simulink model "lon_Input"  (R2016a)
settings: Solver=VariableStepAuto  StartTime=0.0  StopTime=1000  RelTol=1e-3
undefined symbols (not defined in the file): Alon, Blon, Clon, Dlon
settings Model: Creator=Gray  LastModifiedBy=Gray

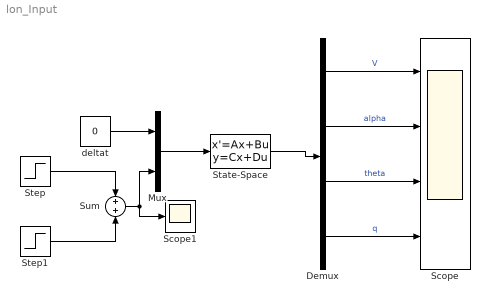
== system lon_Input ==
  Demux : Demux
  Mux : Mux  Inputs=2
  Scope : Scope  NumInputPorts=4
  Scope1 : Scope
  State-Space : StateSpace  A=Alon  B=Blon  C=Clon  D=Dlon  X0=[0 0 0 0]'
  Step : Step  After=2  SampleTime=0
  Step1 : Step  Time=2  After=-2  SampleTime=0
  Sum : Sum
  deltat : Constant  Value=0
  wires:
  State-Space/1 -> Demux/1
  Mux/1 -> State-Space/1
  deltat/1 -> Mux/1
  Demux/1 -> Scope/1  "V"
  Demux/2 -> Scope/2  "alpha"
  Demux/3 -> Scope/3  "theta"
  Demux/4 -> Scope/4  "q"
  Step/1 -> Sum/1
  Sum/1 -> Scope1/1, Mux/2
  Step1/1 -> Sum/2
